simulink model "train_network"  (R2019a)
settings: Solver=VariableStepAuto  StartTime=0.0  StopTime=2400  RelTol=1e-3
values from neighbouring files (symbols this model uses):
  door_opening = [15 15 15 15 15 15 15]    [get_parameters.m]
  train_frequencies = struct    [get_parameters.m]
  travel_times = [ 0       60    0      0      0     0        0 ... (first row only)    [get_parameters.m]
undefined symbols (not defined in the file or in its folder): m, n
(part 1 of 2)
settings Model: SimulationMode=accelerator  OrderedModelArguments=off  Creator=Fredrik Rahm  LastModifiedBy=mawass

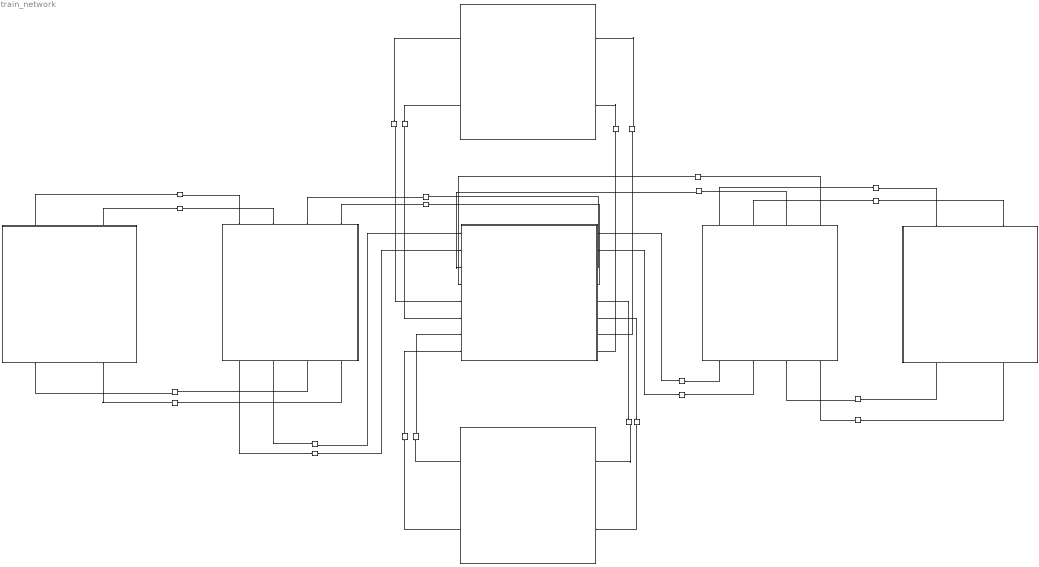
== system train_network ==
  Door signal delay1 : EntityServer  InputPortMessageModes=m  OutputPortMessageModes=m  Capacity=inf  ServiceTimeValue=travel_times(4,5)
  Signal delay10 : EntityServer  InputPortMessageModes=m  OutputPortMessageModes=m  Capacity=inf  ServiceTimeValue=travel_times(4,3)
  Signal delay11 : EntityServer  InputPortMessageModes=m  OutputPortMessageModes=m  Capacity=inf  ServiceTimeValue=travel_times(3,2)
  Signal delay12 : EntityServer  InputPortMessageModes=m  OutputPortMessageModes=m  Capacity=inf  ServiceTimeValue=travel_times(6,3)
  Signal delay14 : EntityServer  InputPortMessageModes=m  OutputPortMessageModes=m  Capacity=inf  ServiceTimeValue=travel_times(7,3)
  Signal delay2 : EntityServer  InputPortMessageModes=m  OutputPortMessageModes=m  Capacity=inf  ServiceTimeValue=travel_times(3,7)
  Signal delay3 : EntityServer  InputPortMessageModes=m  OutputPortMessageModes=m  Capacity=inf  ServiceTimeValue=travel_times(1,2)
  Signal delay4 : EntityServer  InputPortMessageModes=m  OutputPortMessageModes=m  Capacity=inf  ServiceTimeValue=travel_times(2,1)
  Signal delay5 : EntityServer  InputPortMessageModes=m  OutputPortMessageModes=m  Capacity=inf  ServiceTimeValue=travel_times(5,4)
  Signal delay6 : EntityServer  InputPortMessageModes=m  OutputPortMessageModes=m  Capacity=inf  ServiceTimeValue=travel_times(3,6)
  Signal delay8 : EntityServer  InputPortMessageModes=m  OutputPortMessageModes=m  Capacity=inf  ServiceTimeValue=travel_times(2,3)
  Signal delay9 : EntityServer  InputPortMessageModes=m  OutputPortMessageModes=m  Capacity=inf  ServiceTimeValue=travel_times(3,4)
  Station 1 : Subsystem
  Station 1. East. Travelling to Station 2. : EntityServer  InputPortMessageModes=m  OutputPortMessageModes=n,m  Capacity=train_cap  ServiceTimeValue=travel_times(1,2)  NumberEntitiesInBlock=on
      settings: OutputPortMap=o1,o9
  Station 2 : Subsystem
  Station 2. East. Travelling to Station 3. : EntityServer  InputPortMessageModes=m  OutputPortMessageModes=n,m  Capacity=train_cap  ServiceTimeValue=travel_times(2,3)  NumberEntitiesInBlock=on
      settings: OutputPortMap=o1,o9
  Station 2. West. Travelling to Station 1. : EntityServer  InputPortMessageModes=m  OutputPortMessageModes=n,m  Capacity=train_cap  ServiceTimeValue=travel_times(2,1)  NumberEntitiesInBlock=on
      settings: OutputPortMap=o1,o9
  Station 3 : Subsystem
  Station 3. East. Travelling to Station 4. : EntityServer  InputPortMessageModes=m  OutputPortMessageModes=n,m  Capacity=train_cap  ServiceTimeValue=travel_times(3,4)  NumberEntitiesInBlock=on
      settings: OutputPortMap=o1,o9
  Station 3. North. Travelling to Station 6. : EntityServer  InputPortMessageModes=m  OutputPortMessageModes=n,m  Capacity=train_cap  ServiceTimeValue=travel_times(3,6)  NumberEntitiesInBlock=on
      settings: OutputPortMap=o1,o9
  Station 3. West. Travelling to Station 2. : EntityServer  InputPortMessageModes=m  OutputPortMessageModes=n,m  Capacity=train_cap  ServiceTimeValue=travel_times(3,2)  NumberEntitiesInBlock=on
      settings: OutputPortMap=o1,o9
  Station 4 : Subsystem
  Station 4. East. Travelling to Station 5. : EntityServer  InputPortMessageModes=m  OutputPortMessageModes=n,m  Capacity=train_cap  ServiceTimeValue=travel_times(4,5)  NumberEntitiesInBlock=on
      settings: OutputPortMap=o1,o9
  Station 4. West. Travelling to Station 3. : EntityServer  InputPortMessageModes=m  OutputPortMessageModes=n,m  Capacity=train_cap  ServiceTimeValue=travel_times(4,3)  NumberEntitiesInBlock=on
      settings: OutputPortMap=o1,o9
  Station 5 : Subsystem
  Station 5. West. Travelling to Station 4. : EntityServer  InputPortMessageModes=m  OutputPortMessageModes=n,m  Capacity=train_cap  ServiceTimeValue=travel_times(5,4)  NumberEntitiesInBlock=on
      settings: OutputPortMap=o1,o9
  Station 6 : Subsystem
  Station 6. South. Travelling to Station 3. : EntityServer  InputPortMessageModes=m  OutputPortMessageModes=n,m  Capacity=1000  ServiceTimeValue=travel_times(6,3)  NumberEntitiesInBlock=on
      settings: OutputPortMap=o1,o9
  "Station 7 " : Subsystem
  Station 8. South. Travelling to Station 9. : EntityServer  InputPortMessageModes=m  OutputPortMessageModes=n,m  Capacity=train_cap  ServiceTimeValue=travel_times(3,7)  NumberEntitiesInBlock=on
      settings: OutputPortMap=o1,o9
  Station 9. North. Travelling to Station 8. : EntityServer  InputPortMessageModes=m  OutputPortMessageModes=n,m  Capacity=train_cap  ServiceTimeValue=travel_times(7,3)  NumberEntitiesInBlock=on
      settings: OutputPortMap=o1,o9
  wires:
  Station 4. East. Travelling to Station 5./2 -> Station 5/1(People in east)
  Door signal delay1/1 -> Station 5/2(Signal in east)
  Station 5/1(Train out west) -> Station 5. West. Travelling to Station 4./1
  Station 5/2(Signal out west) -> Signal delay5/1
  Station 3/2(Signal East out) -> Signal delay9/1
  Station 5. West. Travelling to Station 4./2 -> Station 4/3(Train in west)
  Signal delay5/1 -> Station 4/4(Signal in west)
  Station 4/1(People east) -> Station 4. East. Travelling to Station 5./1
  Station 4/2(Signal east) -> Door signal delay1/1
  Station 4/3(People west) -> Station 4. West. Travelling to Station 3./1
  Station 1. East. Travelling to Station 2./2 -> Station 2/1(People in east)
  Signal delay3/1 -> Station 2/2(Signal in east)
  Station 3/3(Train West out) -> Station 3. West. Travelling to Station 2./1
  Station 2/2(People out east) -> Station 2. East. Travelling to Station 3./1
  Station 2/3(People out west) -> Station 2. West. Travelling to Station 1./1
  Station 2/4(Signal out west) -> Signal delay4/1
  Station 2. West. Travelling to Station 1./2 -> Station 1/1(Train in west)
  Signal delay4/1 -> Station 1/2(Signal in west)
  Station 1/1(People east) -> Station 1. East. Travelling to Station 2./1
  Station 1/2(Signal East) -> Signal delay3/1
  Station 3/8(Signal North out) -> Signal delay6/1
  Station 8. South. Travelling to Station 9./2 -> "Station 7 "/1(People in south)
  Signal delay2/1 -> "Station 7 "/2(Signal in south)
  "Station 7 "/1(People out north) -> Station 9. North. Travelling to Station 8./1
  "Station 7 "/2(Signal out north) -> Signal delay14/1
  Station 3/7(Train North out) -> Station 3. North. Travelling to Station 6./1
  Station 2. East. Travelling to Station 3./2 -> Station 3/1(Train East in)
  Station 2/1(Signal out east) -> Signal delay8/1
  Signal delay8/1 -> Station 3/2(Signal East in)
  Signal delay9/1 -> Station 4/2(Signal in east)
  Station 3. East. Travelling to Station 4./2 -> Station 4/1(People in east)
  Station 3/1(Train East out) -> Station 3. East. Travelling to Station 4./1
  Station 4. West. Travelling to Station 3./2 -> Station 3/3(Train West in)
  Signal delay10/1 -> Station 3/4(Signal West in)
  Station 4/4(Signal west) -> Signal delay10/1
  Station 3. West. Travelling to Station 2./2 -> Station 2/3(People in west)
  Signal delay11/1 -> Station 2/4(Signal in west)
  Station 3/4(Signal West out) -> Signal delay11/1
  Signal delay12/1 -> Station 3/6(Signal South in)
  Station 6. South. Travelling to Station 3./2 -> Station 3/5(Train South in)
  Signal delay14/1 -> Station 3/8(Signal North in)
  Station 9. North. Travelling to Station 8./2 -> Station 3/7(Train North in)
  Station 3/5(Train South out) -> Station 8. South. Travelling to Station 9./1
  Station 3/6(Signal South out) -> Signal delay2/1
  Station 6/1(Train South) -> Station 6. South. Travelling to Station 3./1
  Station 6/2(Signal south) -> Signal delay12/1
  Signal delay6/1 -> Station 6/2(Signal north)
  Station 3. North. Travelling to Station 6./2 -> Station 6/1(Train north)

== system train_network/Station 1 ==
  Train in west : Inport
  Signal in west : Inport  Port=2
  Add : Sum
  Counting : EntityServer  InputPortMessageModes=m  OutputPortMessageModes=n,m  Capacity=inf  ServiceTimeSource=MATLAB action  ServiceTimeValue=1  ServiceTimeAction=|  NumberEntitiesInBlock=on
      | persistent rngInit;
      | if isempty(rngInit)
      |     seed = 12345;
      |     rng(seed);
      |     rngInit = true;
      | end
      | 
      | % Pattern: Gaussian (normal) distribution
      | % m: Mean, d: Standard deviation
      | m = 40; d = 8;
      | dt = m + d * randn;
      settings: OutputPortMap=o1,o9
  Entity Queue : EntityQueue  InputPortMessageModes=m  OutputPortMessageModes=m  Capacity=50  EntryAction=|
      | coder.extrinsic("get_param");
      | time = double(0);
      | time = get_param("train_network", "SimulationTime");
      | lifetime = time - entity.Timer;
      | 
      | coder.extrinsic("evalin");
      | evalin("base", sprintf("lifetimes_1(1,end+1) = %f; lifetimes_1(2,end) = %f;", lifetime, entity.StartStation));
      settings: OutputPortMap=o5
  Entity Terminator : EntityTerminator  InputPortMessageModes=m
  Station 1 - East : Subsystem
  Station 1 - West : Subsystem
  Station 1. People arriving. : EntityGenerator  OutputPortMessageModes=m  TimeSource=MATLAB action  IntergenerationTimeAction=|  GenerateAction=|  AttributeName=EndStation|Timer|StartStation  AttributeInitialValue=0|0|1  EntityType=Structured  EntityTypeName=Inbound
      | persistent rngInit;
      | if isempty(rngInit)
      |     seed = 173499;
      |     rng(seed);
      |     rngInit = true;
      | end
      | 
      | % Pattern: Exponential distribution
      | mu = lambda(1);
      | dt = -mu * log(1 - rand());
      | persistent rngInit;
      | if isempty(rngInit)
      |     seed = 12345;
      |     rng(seed);
      |     rngInit = true;
      | end
      | 
      | % Pattern: Arbitrary discrete distribution
      | % V: Value vector
      | % P: Probability vector
      | V = [1 2 3 4 5 6 7];
      | Ps = P(entity.StartStation,:);
      | entity.EndStation = randsample(V, 1, true, Ps);
      | 
      | coder.extrinsic("get_param");
      | entity.Timer = get_param("train_network", "SimulationTime");
  People east : Outport
  Signal East : Outport  Port=2
  wires:
  Train in west/1 -> Station 1 - West/1(Train in)
  Station 1 - East/2(Signal) -> Signal East/1
  Signal in west/1 -> Station 1 - West/2(Door control)
  Station 1. People arriving./1 -> Station 1 - East/1(Inport)
  Station 1 - East/1(Train) -> People east/1
  Counting/2 -> Entity Terminator/1
  Counting/1 -> Add/1
  Entity Queue/1 -> Counting/1
  Station 1 - West/1("Unboard ") -> Entity Queue/1
  Station 1 - East/3(Peopleplatform number) -> Add/2

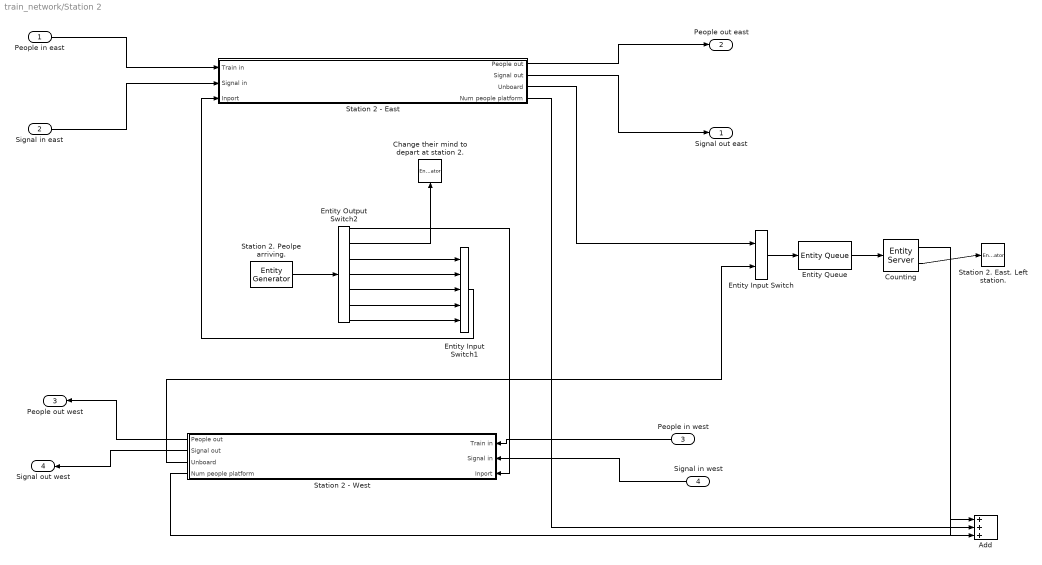
== system train_network/Station 2 ==
  People in east : Inport
  Signal in east : Inport  Port=2
  People in west : Inport  Port=3
  Signal in west : Inport  Port=4
  Add : Sum  Inputs=+++
  Change their mind to depart at station 2. : EntityTerminator  InputPortMessageModes=m
  Counting : EntityServer  InputPortMessageModes=m  OutputPortMessageModes=n,m  Capacity=inf  ServiceTimeSource=MATLAB action  ServiceTimeValue=1  ServiceTimeAction=|  NumberEntitiesInBlock=on
      | persistent rngInit;
      | if isempty(rngInit)
      |     seed = 12345;
      |     rng(seed);
      |     rngInit = true;
      | end
      | 
      | % Pattern: Gaussian (normal) distribution
      | % m: Mean, d: Standard deviation
      | m = 40; d = 8;
      | dt = m + d * randn;
      settings: OutputPortMap=o1,o9
  Entity Input Switch : EntityInputSwitch  InputPortMessageModes=m,m  OutputPortMessageModes=m
  Entity Input Switch1 : EntityInputSwitch  InputPortMessageModes=m,m,m,m,m  OutputPortMessageModes=m  NumberInputPorts=5
      settings: InputPortMap=u1,u2,u3,u4,u5
  Entity Output Switch2 : EntityOutputSwitch  InputPortMessageModes=m  OutputPortMessageModes=m,m,m,m,m,m,m  NumberOutputPorts=7  SwitchingCriterion=From attribute  SwitchAttributeName=EndStation
      settings: OutputPortMap=o0,o1,o2,o3,o4,o5,o6
  Entity Queue : EntityQueue  InputPortMessageModes=m  OutputPortMessageModes=m  Capacity=50  EntryAction=|
      | coder.extrinsic("get_param");
      | time = double(0);
      | time = get_param("train_network", "SimulationTime");
      | lifetime = time - entity.Timer;
      | 
      | coder.extrinsic("evalin");
      | evalin("base", sprintf("lifetimes_2(1,end+1) = %f; lifetimes_2(2,end) = %f;", lifetime, entity.StartStation));
      settings: OutputPortMap=o5
  Station 2 - East : Subsystem
  Station 2 - West : Subsystem
  Station 2. East. Left station. : EntityTerminator  InputPortMessageModes=m  NumberEntitiesArrived=on
      settings: OutputPortMap=o0
  Station 2. Peolpe arriving. : EntityGenerator  OutputPortMessageModes=m  TimeSource=MATLAB action  IntergenerationTimeAction=|  GenerateAction=|  AttributeName=EndStation|Timer|StartStation  AttributeInitialValue=0|0|2  EntityType=Structured  EntityTypeName=Inbound
      | persistent rngInit;
      | if isempty(rngInit)
      |     seed = 173499;
      |     rng(seed);
      |     rngInit = true;
      | end
      | 
      | % Pattern: Exponential distribution
      | mu = lambda(2);
      | dt = -mu * log(1 - rand());
      | persistent rngInit;
      | if isempty(rngInit)
      |     seed = 12345;
      |     rng(seed);
      |     rngInit = true;
      | end
      | 
      | % Pattern: Arbitrary discrete distribution
      | % V: Value vector
      | % P: Probability vector
      | V = [1 2 3 4 5 6 7];
      | Ps = P(entity.StartStation,:);
      | entity.EndStation = randsample(V, 1, true, Ps);
      | 
      | coder.extrinsic("get_param");
      | entity.Timer = get_param("train_network", "SimulationTime");
  Signal out east : Outport
  People out east : Outport  Port=2
  People out west : Outport  Port=3
  Signal out west : Outport  Port=4
  wires:
  Signal in west/1 -> Station 2 - West/2(Signal in)
  Entity Input Switch1/1 -> Station 2 - East/3(Inport)
  Entity Output Switch2/1 -> Station 2 - West/3(Inport)
  Station 2 - West/1(People out) -> People out west/1
  People in east/1 -> Station 2 - East/1(Train in)
  Station 2 - East/2(Signal out) -> Signal out east/1
  Station 2 - East/1(People out) -> People out east/1
  People in west/1 -> Station 2 - West/1(Train in)
  Station 2 - West/2(Signal out) -> Signal out west/1
  Signal in east/1 -> Station 2 - East/2(Signal in)
  Station 2. Peolpe arriving./1 -> Entity Output Switch2/1
  Entity Output Switch2/7 -> Entity Input Switch1/5
  Entity Output Switch2/6 -> Entity Input Switch1/4
  Entity Output Switch2/5 -> Entity Input Switch1/3
  Entity Output Switch2/4 -> Entity Input Switch1/2
  Entity Output Switch2/3 -> Entity Input Switch1/1
  Entity Output Switch2/2 -> Change their mind to depart at station 2./1
  Station 2 - East/3(Unboard) -> Entity Input Switch/1
  Station 2 - West/3(Unboard) -> Entity Input Switch/2
  Station 2 - West/4(Num people platform) -> Add/3
  Counting/2 -> Station 2. East. Left station./1
  Counting/1 -> Add/1
  Station 2 - East/4("Num people platform ") -> Add/2
  Entity Input Switch/1 -> Entity Queue/1
  Entity Queue/1 -> Counting/1

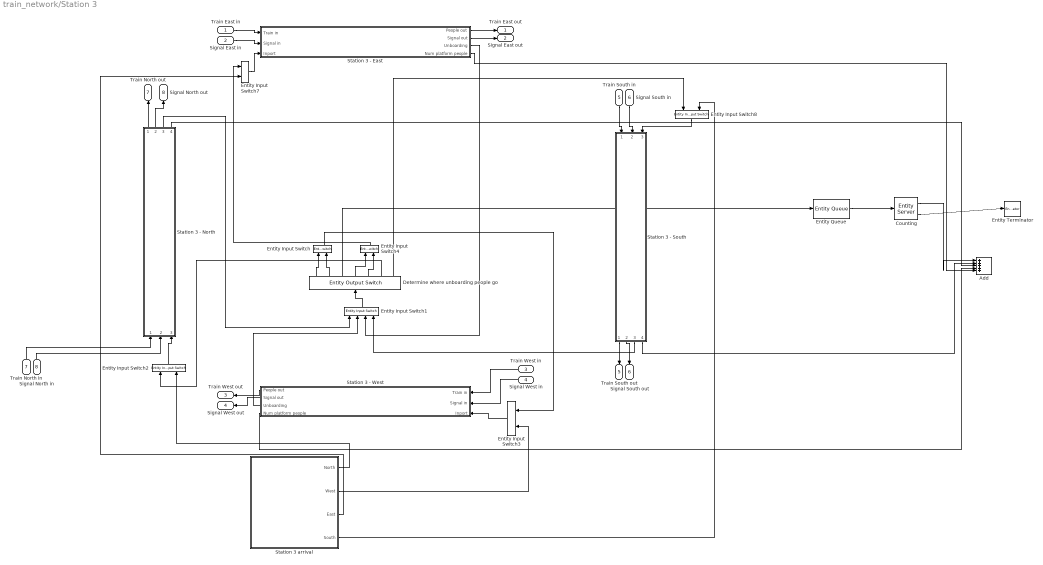
== system train_network/Station 3 ==
  Train East in : Inport
  Signal East in : Inport  Port=2
  Train West in : Inport  Port=3
  Signal West in : Inport  Port=4
  Train South in : Inport  Port=5
  Signal South in : Inport  Port=6
  Train North in : Inport  Port=7
  Signal North in : Inport  Port=8
  Add : Sum  Inputs=+++++
  Counting : EntityServer  InputPortMessageModes=m  OutputPortMessageModes=n,m  Capacity=inf  ServiceTimeSource=MATLAB action  ServiceTimeValue=1  ServiceTimeAction=|  NumberEntitiesInBlock=on
      | persistent rngInit;
      | if isempty(rngInit)
      |     seed = 12345;
      |     rng(seed);
      |     rngInit = true;
      | end
      | 
      | % Pattern: Gaussian (normal) distribution
      | % m: Mean, d: Standard deviation
      | m = 40; d = 8;
      | dt = m + d * randn;
      settings: OutputPortMap=o1,o9
  Determine where unboarding people go : EntityOutputSwitch  InputPortMessageModes=m  OutputPortMessageModes=m,m,m,m,m,m,m  NumberOutputPorts=7  SwitchingCriterion=From attribute  SwitchAttributeName=EndStation
      settings: OutputPortMap=o0,o1,o2,o3,o4,o5,o6
  Entity Input Switch{,2..4,7..8} (6 alike) : EntityInputSwitch  InputPortMessageModes=m,m  OutputPortMessageModes=m
  Entity Input Switch1 : EntityInputSwitch  InputPortMessageModes=m,m,m,m  OutputPortMessageModes=m  NumberInputPorts=4
      settings: InputPortMap=u1,u2,u3,u4
  Entity Queue : EntityQueue  InputPortMessageModes=m  OutputPortMessageModes=m  Capacity=50  EntryAction=|
      | coder.extrinsic("get_param");
      | time = double(0);
      | time = get_param("train_network", "SimulationTime");
      | lifetime = time - entity.Timer;
      | 
      | coder.extrinsic("evalin");
      | evalin("base", sprintf("lifetimes_3(1,end+1) = %f; lifetimes_3(2,end) = %f;", lifetime, entity.StartStation));
      settings: OutputPortMap=o5
  Entity Terminator : EntityTerminator  InputPortMessageModes=m
  Station 3 - East : Subsystem
  Station 3 - North : Subsystem
  Station 3 - South : Subsystem
  Station 3 - West : Subsystem
  Station 3 arrival : Subsystem
  Train East out : Outport
  Signal East out : Outport  Port=2
  Train West out : Outport  Port=3
  Signal West out : Outport  Port=4
  Train South out : Outport  Port=5
  Signal South out : Outport  Port=6
  Train North out : Outport  Port=7
  Signal North out : Outport  Port=8
  wires:
  Train East in/1 -> Station 3 - East/1(Train in)
  Station 3 - East/1(People out) -> Train East out/1
  Station 3 - East/2(Signal out) -> Signal East out/1
  Signal East in/1 -> Station 3 - East/2(Signal in)
  Station 3 - West/1(People out) -> Train West out/1
  Station 3 - West/2(Signal out) -> Signal West out/1
  Train West in/1 -> Station 3 - West/1(Train in)
  Signal West in/1 -> Station 3 - West/2(Signal in)
  Signal South in/1 -> Station 3 - South/2(Signal in)
  Train South in/1 -> Station 3 - South/1(Train in)
  Station 3 - South/2(Signal out) -> Signal South out/1
  Station 3 - South/1(People out) -> Train South out/1
  Signal North in/1 -> Station 3 - North/2(Signal in)
  Train North in/1 -> Station 3 - North/1(Train in)
  Station 3 - North/1(People out) -> Train North out/1
  Station 3 - North/2(Signal out) -> Signal North out/1
  Station 3 arrival/2(West) -> Entity Input Switch3/2
  Station 3 arrival/3(East) -> Entity Input Switch7/2
  Station 3 arrival/4(South) -> Entity Input Switch8/2
  Station 3 - North/3(Unboarding) -> Entity Input Switch1/1
  Station 3 - South/3(Unboarding) -> Entity Input Switch1/4
  Station 3 - West/3(Unboarding) -> Entity Input Switch1/2
  Station 3 - East/3(Unboarding) -> Entity Input Switch1/3
  Entity Input Switch2/1 -> Station 3 - North/3(Inport)
  Station 3 arrival/1(North) -> Entity Input Switch2/2
  Entity Input Switch1/1 -> Determine where unboarding people go/1
  Determine where unboarding people go/1 -> Entity Input Switch/1
  Determine where unboarding people go/2 -> Entity Input Switch/2
  Entity Input Switch3/1 -> Station 3 - West/3(Inport)
  Entity Input Switch/1 -> Entity Input Switch3/1
  Determine where unboarding people go/4 -> Entity Input Switch4/1
  Determine where unboarding people go/5 -> Entity Input Switch4/2
  Entity Input Switch7/1 -> Station 3 - East/3(Inport)
  Entity Input Switch4/1 -> Entity Input Switch7/1
  Entity Input Switch8/1 -> Station 3 - South/3(Inport)
  Determine where unboarding people go/6 -> Entity Input Switch2/1
  Determine where unboarding people go/7 -> Entity Input Switch8/1
  Counting/2 -> Entity Terminator/1
  Counting/1 -> Add/1
  Determine where unboarding people go/3 -> Entity Queue/1
  Entity Queue/1 -> Counting/1
  Station 3 - South/4(Num platform people) -> Add/2
  Station 3 - West/4(Num platform people) -> Add/4
  Station 3 - North/4(Num platform people) -> Add/3
  Station 3 - East/4(Num platform people) -> Add/5

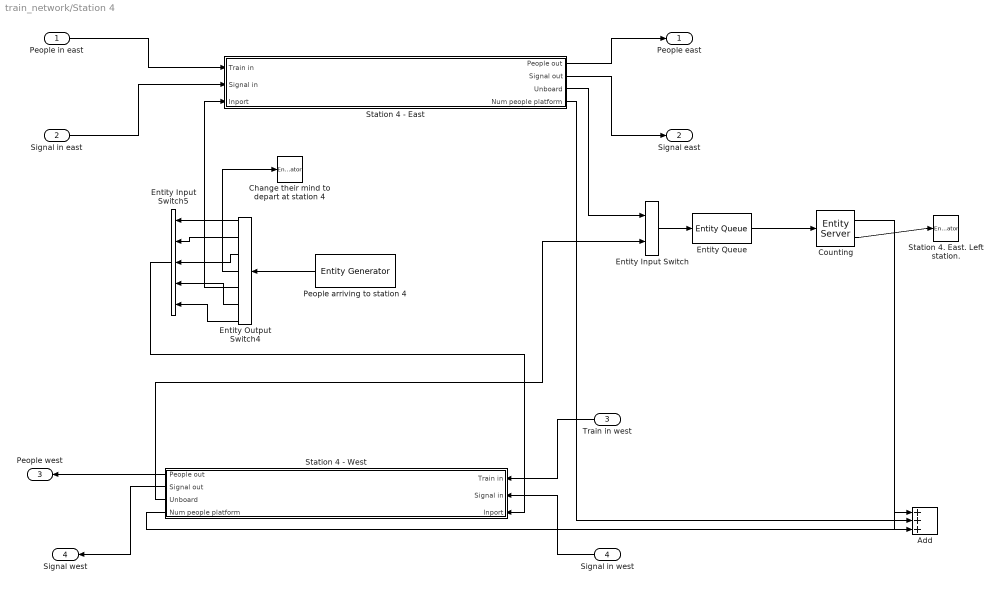
== system train_network/Station 4 ==
  People in east : Inport
  Signal in east : Inport  Port=2
  Train in west : Inport  Port=3
  Signal in west : Inport  Port=4
  Add : Sum  Inputs=+++
  Change their mind to depart at station 4 : EntityTerminator  InputPortMessageModes=m
  Counting : EntityServer  InputPortMessageModes=m  OutputPortMessageModes=n,m  Capacity=inf  ServiceTimeSource=MATLAB action  ServiceTimeValue=1  ServiceTimeAction=|  NumberEntitiesInBlock=on
      | persistent rngInit;
      | if isempty(rngInit)
      |     seed = 12345;
      |     rng(seed);
      |     rngInit = true;
      | end
      | 
      | % Pattern: Gaussian (normal) distribution
      | % m: Mean, d: Standard deviation
      | m = 40; d = 8;
      | dt = m + d * randn;
      settings: OutputPortMap=o1,o9
  Entity Input Switch : EntityInputSwitch  InputPortMessageModes=m,m  OutputPortMessageModes=m
  Entity Input Switch5 : EntityInputSwitch  InputPortMessageModes=m,m,m,m,m  OutputPortMessageModes=m  NumberInputPorts=5
      settings: InputPortMap=u1,u2,u3,u4,u5
  Entity Output Switch4 : EntityOutputSwitch  InputPortMessageModes=m  OutputPortMessageModes=m,m,m,m,m,m,m  NumberOutputPorts=7  SwitchingCriterion=From attribute  SwitchAttributeName=EndStation
      settings: OutputPortMap=o0,o1,o2,o3,o4,o5,o6
  Entity Queue : EntityQueue  InputPortMessageModes=m  OutputPortMessageModes=m  Capacity=50  EntryAction=|
      | coder.extrinsic("get_param");
      | time = double(0);
      | time = get_param("train_network", "SimulationTime");
      | lifetime = time - entity.Timer;
      | 
      | coder.extrinsic("evalin");
      | evalin("base", sprintf("lifetimes_4(1,end+1) = %f; lifetimes_4(2,end) = %f;", lifetime, entity.StartStation));
      settings: OutputPortMap=o5
  People arriving to station 4 : EntityGenerator  OutputPortMessageModes=m  TimeSource=MATLAB action  IntergenerationTimeAction=|  GenerateAction=|  AttributeName=EndStation|Timer|StartStation  AttributeInitialValue=0|1|4  EntityType=Structured  EntityTypeName=Inbound
      | persistent rngInit;
      | if isempty(rngInit)
      |     seed = 173499;
      |     rng(seed);
      |     rngInit = true;
      | end
      | 
      | % Pattern: Exponential distribution
      | mu = lambda(4);
      | dt = -mu * log(1 - rand());
      | persistent rngInit;
      | if isempty(rngInit)
      |     seed = 12345;
      |     rng(seed);
      |     rngInit = true;
      | end
      | 
      | % Pattern: Arbitrary discrete distribution
      | % V: Value vector
      | % P: Probability vector
      | V = [1 2 3 4 5 6 7];
      | Ps = P(entity.StartStation,:);
      | entity.EndStation = randsample(V, 1, true, Ps);
      | 
      | coder.extrinsic("get_param");
      | entity.Timer = get_param("train_network", "SimulationTime");
  Station 4 - East : Subsystem
  Station 4 - West : Subsystem
  Station 4. East. Left station. : EntityTerminator  InputPortMessageModes=m
  People east : Outport
  Signal east : Outport  Port=2
  People west : Outport  Port=3
  Signal west : Outport  Port=4
  wires:
  Entity Input Switch5/1 -> Station 4 - West/3(Inport)
  Signal in west/1 -> Station 4 - West/2(Signal in)
  Signal in east/1 -> Station 4 - East/2(Signal in)
  Entity Output Switch4/4 -> Change their mind to depart at station 4/1
  Station 4 - West/1(People out) -> People west/1
  Station 4 - West/2(Signal out) -> Signal west/1
  People in east/1 -> Station 4 - East/1(Train in)
  Entity Output Switch4/5 -> Station 4 - East/3(Inport)
  Station 4 - East/1(People out) -> People east/1
  Train in west/1 -> Station 4 - West/1(Train in)
  Station 4 - East/2(Signal out) -> Signal east/1
  People arriving to station 4/1 -> Entity Output Switch4/1
  Station 4 - East/3(Unboard) -> Entity Input Switch/1
  Station 4 - West/3(Unboard) -> Entity Input Switch/2
  Entity Output Switch4/1 -> Entity Input Switch5/1
  Entity Output Switch4/2 -> Entity Input Switch5/2
  Entity Output Switch4/3 -> Entity Input Switch5/3
  Entity Output Switch4/6 -> Entity Input Switch5/4
  Entity Output Switch4/7 -> Entity Input Switch5/5
  Entity Queue/1 -> Counting/1
  Counting/2 -> Station 4. East. Left station./1
  Counting/1 -> Add/1
  Entity Input Switch/1 -> Entity Queue/1
  Station 4 - West/4(Num people platform) -> Add/3
  Station 4 - East/4(Num people platform) -> Add/2

== system train_network/Station 5 ==
  People in east : Inport
  Signal in east : Inport  Port=2
  Add : Sum
  Counting : EntityServer  InputPortMessageModes=m  OutputPortMessageModes=n,m  Capacity=inf  ServiceTimeSource=MATLAB action  ServiceTimeValue=1  ServiceTimeAction=|  NumberEntitiesInBlock=on
      | persistent rngInit;
      | if isempty(rngInit)
      |     seed = 12345;
      |     rng(seed);
      |     rngInit = true;
      | end
      | 
      | % Pattern: Gaussian (normal) distribution
      | % m: Mean, d: Standard deviation
      | m = 40; d = 8;
      | dt = m + d * randn;
      settings: OutputPortMap=o1,o9
  Entity Queue : EntityQueue  InputPortMessageModes=m  OutputPortMessageModes=m  Capacity=50  EntryAction=|
      | coder.extrinsic("get_param");
      | time = double(0);
      | time = get_param("train_network", "SimulationTime");
      | lifetime = time - entity.Timer;
      | 
      | coder.extrinsic("evalin");
      | evalin("base", sprintf("lifetimes_5(1,end+1) = %f; lifetimes_5(2,end) = %f;", lifetime, entity.StartStation));
      settings: OutputPortMap=o5
  Entity Terminator : EntityTerminator  InputPortMessageModes=m
  People arriving to station 5. : EntityGenerator  OutputPortMessageModes=m  TimeSource=MATLAB action  IntergenerationTimeAction=|  GenerateAction=|  AttributeName=EndStation|Timer|StartStation  AttributeInitialValue=0|0|5  EntityType=Structured  EntityTypeName=Inbound
      | persistent rngInit;
      | if isempty(rngInit)
      |     seed = 173499;
      |     rng(seed);
      |     rngInit = true;
      | end
      | 
      | % Pattern: Exponential distribution
      | mu = lambda(5);
      | dt = -mu * log(1 - rand());
      | persistent rngInit;
      | if isempty(rngInit)
      |     seed = 12345;
      |     rng(seed);
      |     rngInit = true;
      | end
      | 
      | % Pattern: Arbitrary discrete distribution
      | % V: Value vector
      | % P: Probability vector
      | V = [1 2 3 4 5 6 7];
      | Ps = P(entity.StartStation,:);
      | entity.EndStation = randsample(V, 1, true, Ps);
      | 
      | coder.extrinsic("get_param");
      | entity.Timer = get_param("train_network", "SimulationTime");
  Station 5 - East : Subsystem
  Station 5 - West : Subsystem
  Train out west : Outport
  Signal out west : Outport  Port=2
  wires:
  Station 5 - West/2(Signal) -> Signal out west/1
  Station 5 - West/1(Train) -> Train out west/1
  Signal in east/1 -> Station 5 - East/2(Door control)
  People in east/1 -> Station 5 - East/1(Train in)
  Entity Queue/1 -> Counting/1
  Counting/2 -> Entity Terminator/1
  Counting/1 -> Add/1
  Station 5 - East/1("Unboard ") -> Entity Queue/1
  Station 5 - West/3(Platform number people) -> Add/2
  People arriving to station 5./1 -> Station 5 - West/1(Inport)

== system train_network/Station 6 ==
  Train north : Inport
  Signal north : Inport  Port=2
  Add : Sum
  Counting : EntityServer  InputPortMessageModes=m  OutputPortMessageModes=n,m  Capacity=inf  ServiceTimeSource=MATLAB action  ServiceTimeValue=1  ServiceTimeAction=|  NumberEntitiesInBlock=on
      | persistent rngInit;
      | if isempty(rngInit)
      |     seed = 12345;
      |     rng(seed);
      |     rngInit = true;
      | end
      | 
      | % Pattern: Gaussian (normal) distribution
      | % m: Mean, d: Standard deviation
      | m = 40; d = 8;
      | dt = m + d * randn;
      settings: OutputPortMap=o1,o9
  Entity Queue : EntityQueue  InputPortMessageModes=m  OutputPortMessageModes=m  Capacity=50  EntryAction=|
      | coder.extrinsic("get_param");
      | time = double(0);
      | time = get_param("train_network", "SimulationTime");
      | lifetime = time - entity.Timer;
      | 
      | coder.extrinsic("evalin");
      | evalin("base", sprintf("lifetimes_6(1,end+1) = %f; lifetimes_6(2,end) = %f;", lifetime, entity.StartStation));
      settings: OutputPortMap=o5
  Entity Terminator : EntityTerminator  InputPortMessageModes=m
  People arriving to station 6. : EntityGenerator  OutputPortMessageModes=m  TimeSource=MATLAB action  IntergenerationTimeAction=|  GenerateAction=|  AttributeName=EndStation|Timer|StartStation  AttributeInitialValue=0|0|6  EntityType=Structured  EntityTypeName=Inbound
      | persistent rngInit;
      | if isempty(rngInit)
      |     seed = 173499;
      |     rng(seed);
      |     rngInit = true;
      | end
      | 
      | % Pattern: Exponential distribution
      | mu = lambda(6);
      | dt = -mu * log(1 - rand());
      | persistent rngInit;
      | if isempty(rngInit)
      |     seed = 12345;
      |     rng(seed);
      |     rngInit = true;
      | end
      | 
      | % Pattern: Arbitrary discrete distribution
      | % V: Value vector
      | % P: Probability vector
      | V = [1 2 3 4 5 6 7];
      | Ps = P(entity.StartStation,:);
      | entity.EndStation = randsample(V, 1, true, Ps);
      | 
      | coder.extrinsic("get_param");
      | entity.Timer = get_param("train_network", "SimulationTime");
  Station 6 - North : Subsystem
  Station 6 - South : Subsystem
  Train South : Outport
  Signal south : Outport  Port=2
  wires:
  People arriving to station 6./1 -> Station 6 - South/1(Inport)
  Station 6 - South/2(Signal) -> Signal south/1
  Station 6 - South/1(Train) -> Train South/1
  Signal north/1 -> Station 6 - North/2(Door control)
  Train north/1 -> Station 6 - North/1(Train in)
  Counting/2 -> Entity Terminator/1
  Counting/1 -> Add/1
  Station 6 - North/1(Unboard) -> Entity Queue/1
  Entity Queue/1 -> Counting/1
  Station 6 - South/3("People on platform ") -> Add/2

== system train_network/Station 7  ==
  People in south : Inport
  Signal in south : Inport  Port=2
  Add : Sum
  Counting : EntityServer  InputPortMessageModes=m  OutputPortMessageModes=n,m  Capacity=inf  ServiceTimeSource=MATLAB action  ServiceTimeValue=1  ServiceTimeAction=|  NumberEntitiesInBlock=on
      | persistent rngInit;
      | if isempty(rngInit)
      |     seed = 12345;
      |     rng(seed);
      |     rngInit = true;
      | end
      | 
      | % Pattern: Gaussian (normal) distribution
      | % m: Mean, d: Standard deviation
      | m = 40; d = 8;
      | dt = m + d * randn;
      settings: OutputPortMap=o1,o9
  Entity Queue : EntityQueue  InputPortMessageModes=m  OutputPortMessageModes=m  Capacity=50  EntryAction=|
      | coder.extrinsic("get_param");
      | time = double(0);
      | time = get_param("train_network", "SimulationTime");
      | lifetime = time - entity.Timer;
      | 
      | coder.extrinsic("evalin");
      | evalin("base", sprintf("lifetimes_7(1,end+1) = %f; lifetimes_7(2,end) = %f;", lifetime, entity.StartStation));
      settings: OutputPortMap=o5
  Entity Terminator : EntityTerminator  InputPortMessageModes=m
  People arriving to station 7 : EntityGenerator  OutputPortMessageModes=m  TimeSource=MATLAB action  IntergenerationTimeAction=|  GenerateAction=|  AttributeName=EndStation|Timer|StartStation  AttributeInitialValue=0|0|7  EntityType=Structured  EntityTypeName=Inbound
      | persistent rngInit;
      | if isempty(rngInit)
      |     seed = 173499;
      |     rng(seed);
      |     rngInit = true;
      | end
      | 
      | % Pattern: Exponential distribution
      | mu = lambda(7);
      | dt = -mu * log(1 - rand());
      | persistent rngInit;
      | if isempty(rngInit)
      |     seed = 12345;
      |     rng(seed);
      |     rngInit = true;
      | end
      | 
      | % Pattern: Arbitrary discrete distribution
      | % V: Value vector
      | % P: Probability vector
      | V = [1 2 3 4 5 6 7];
      | Ps = P(entity.StartStation,:);
      | entity.EndStation = randsample(V, 1, true, Ps);
      | 
      | coder.extrinsic("get_param");
      | entity.Timer = get_param("train_network", "SimulationTime");
  Station 7 - North : Subsystem
  Station 7 - South : Subsystem
  People out north : Outport
  Signal out north : Outport  Port=2
  wires:
  Signal in south/1 -> Station 7 - South/2(Door control)
  Station 7 - North/2(Signal) -> Signal out north/1
  Station 7 - North/1(Train) -> People out north/1
  People arriving to station 7/1 -> Station 7 - North/1(Inport)
  People in south/1 -> Station 7 - South/1(Train in)
  Counting/2 -> Entity Terminator/1
  Station 7 - South/1(Out1) -> Entity Queue/1
  Entity Queue/1 -> Counting/1
  Counting/1 -> Add/2
  Station 7 - North/3("Num people platform ") -> Add/1

== system train_network/Station 1/Station 1 - East ==
  Inport : Inport
  Departure blocking : EntityGate  InputPortMessageModes=m,m  OutputPortMessageModes=m
  Door controller : Subsystem
  "Station 1, East Train arrives1" : EntityGate  InputPortMessageModes=m,m  OutputPortMessageModes=m
  Station 1. East. People in train while boarding. : EntityServer  InputPortMessageModes=m  OutputPortMessageModes=m  Capacity=train_cap  ServiceTimeValue=0
  Station 1. East. Platform. : EntityQueue  InputPortMessageModes=m  OutputPortMessageModes=n,m  Capacity=inf  NumberEntitiesInBlock=on
      settings: OutputPortMap=o1,o5
  Train : Outport
  Signal : Outport  Port=2
  Peopleplatform number : Outport  Port=3
  wires:
  Station 1. East. Platform./2 -> "Station 1, East Train arrives1"/2
  "Station 1, East Train arrives1"/1 -> Station 1. East. People in train while boarding./1
  Station 1. East. People in train while boarding./1 -> Departure blocking/2
  Departure blocking/1 -> Train/1
  Door controller/1(Next station) -> Signal/1
  Door controller/2(Departure) -> Departure blocking/1
  Door controller/3(Train door) -> "Station 1, East Train arrives1"/1
  Inport/1 -> Station 1. East. Platform./1
  Station 1. East. Platform./1 -> Peopleplatform number/1

== system train_network/Station 1/Station 1 - West ==
  Train in : Inport
  Door control : Inport  Port=2
  " " : EntityGate  InputPortMessageModes=m,m  OutputPortMessageModes=m
  "Unboard " : Outport
  wires:
  Door control/1 -> " "/1
  Train in/1 -> " "/2
  " "/1 -> "Unboard "/1

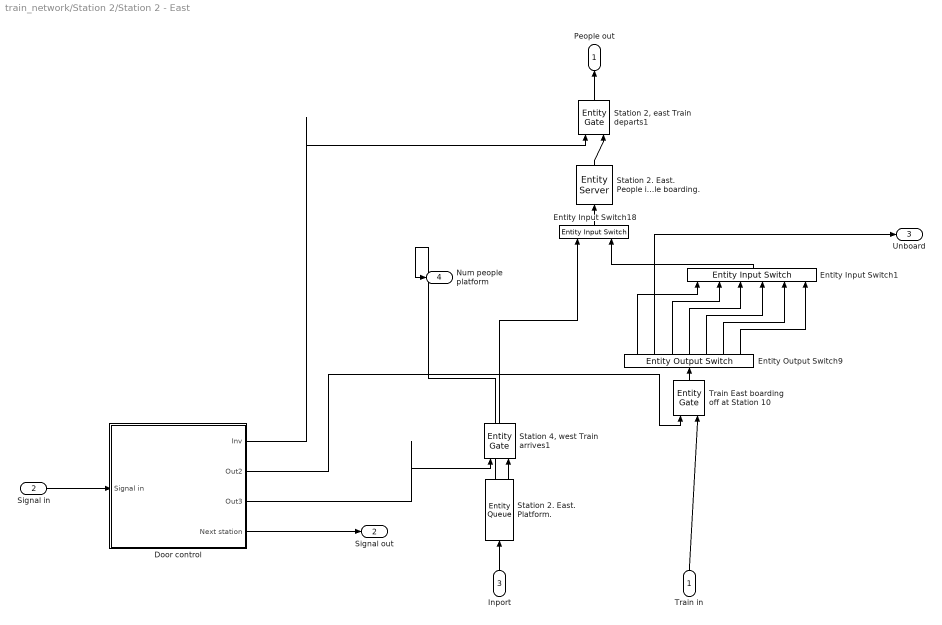
== system train_network/Station 2/Station 2 - East ==
  Train in : Inport
  Signal in : Inport  Port=2
  Inport : Inport  Port=3
  Door control : Subsystem
  Entity Input Switch1 : EntityInputSwitch  InputPortMessageModes=m,m,m,m,m,m  OutputPortMessageModes=m  NumberInputPorts=6
      settings: InputPortMap=u1,u2,u3,u4,u5,u6
  Entity Input Switch18 : EntityInputSwitch  InputPortMessageModes=m,m  OutputPortMessageModes=m
  Entity Output Switch9 : EntityOutputSwitch  InputPortMessageModes=m  OutputPortMessageModes=m,m,m,m,m,m,m  NumberOutputPorts=7  SwitchingCriterion=From attribute  SwitchAttributeName=EndStation
      settings: OutputPortMap=o0,o1,o2,o3,o4,o5,o6
  "Station 2, east Train departs1" : EntityGate  InputPortMessageModes=m,m  OutputPortMessageModes=m
  Station 2. East. People in train while boarding. : EntityServer  InputPortMessageModes=m  OutputPortMessageModes=m  Capacity=train_cap  ServiceTimeValue=0
  "Station 2. East. Platform. " : EntityQueue  InputPortMessageModes=m  OutputPortMessageModes=n,m  Capacity=inf  NumberEntitiesInBlock=on
      settings: OutputPortMap=o1,o5
  "Station 4, west Train arrives1" : EntityGate  InputPortMessageModes=m,m  OutputPortMessageModes=m
  Train East boarding off at Station 10 : EntityGate  InputPortMessageModes=m,m  OutputPortMessageModes=m
  People out : Outport
  Signal out : Outport  Port=2
  Unboard : Outport  Port=3
  "Num people platform " : Outport  Port=4
  wires:
  Train East boarding off at Station 10/1 -> Entity Output Switch9/1
  Inport/1 -> "Station 2. East. Platform. "/1
  Entity Input Switch18/1 -> Station 2. East. People in train while boarding./1
  Station 2. East. People in train while boarding./1 -> "Station 2, east Train departs1"/2
  Train in/1 -> Train East boarding off at Station 10/2
  "Station 2, east Train departs1"/1 -> People out/1
  "Station 2. East. Platform. "/2 -> "Station 4, west Train arrives1"/2
  Entity Output Switch9/1 -> Entity Input Switch1/1
  Entity Output Switch9/2 -> Unboard/1
  "Station 4, west Train arrives1"/1 -> Entity Input Switch18/1
  Door control/1(Inv) -> "Station 2, east Train departs1"/1
  Signal in/1 -> Door control/1(Signal in)
  Door control/4(Next station) -> Signal out/1
  Door control/2(Out2) -> Train East boarding off at Station 10/1
  Door control/3(Out3) -> "Station 4, west Train arrives1"/1
  Entity Output Switch9/3 -> Entity Input Switch1/2
  Entity Output Switch9/4 -> Entity Input Switch1/3
  Entity Output Switch9/5 -> Entity Input Switch1/4
  Entity Output Switch9/6 -> Entity Input Switch1/5
  Entity Output Switch9/7 -> Entity Input Switch1/6
  Entity Input Switch1/1 -> Entity Input Switch18/2
  "Station 2. East. Platform. "/1 -> "Num people platform "/1

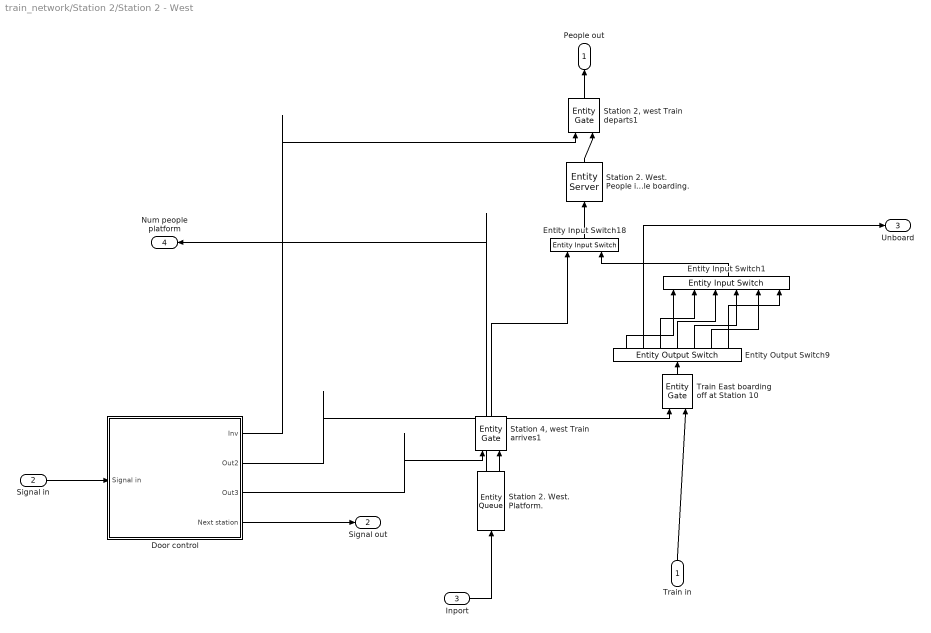
== system train_network/Station 2/Station 2 - West ==
  Train in : Inport
  Signal in : Inport  Port=2
  Inport : Inport  Port=3
  Door control : Subsystem
  Entity Input Switch1 : EntityInputSwitch  InputPortMessageModes=m,m,m,m,m,m  OutputPortMessageModes=m  NumberInputPorts=6
      settings: InputPortMap=u1,u2,u3,u4,u5,u6
  Entity Input Switch18 : EntityInputSwitch  InputPortMessageModes=m,m  OutputPortMessageModes=m
  Entity Output Switch9 : EntityOutputSwitch  InputPortMessageModes=m  OutputPortMessageModes=m,m,m,m,m,m,m  NumberOutputPorts=7  SwitchingCriterion=From attribute  SwitchAttributeName=EndStation
      settings: OutputPortMap=o0,o1,o2,o3,o4,o5,o6
  "Station 2, west Train departs1" : EntityGate  InputPortMessageModes=m,m  OutputPortMessageModes=m
  Station 2. West. People in train while boarding. : EntityServer  InputPortMessageModes=m  OutputPortMessageModes=m  Capacity=train_cap  ServiceTimeValue=0
  Station 2. West. Platform. : EntityQueue  InputPortMessageModes=m  OutputPortMessageModes=n,m  Capacity=inf  NumberEntitiesInBlock=on
      settings: OutputPortMap=o1,o5
  "Station 4, west Train arrives1" : EntityGate  InputPortMessageModes=m,m  OutputPortMessageModes=m
  Train East boarding off at Station 10 : EntityGate  InputPortMessageModes=m,m  OutputPortMessageModes=m
  People out : Outport
  Signal out : Outport  Port=2
  Unboard : Outport  Port=3
  Num people platform : Outport  Port=4
  wires:
  Inport/1 -> Station 2. West. Platform./1
  Entity Input Switch18/1 -> Station 2. West. People in train while boarding./1
  Station 2. West. People in train while boarding./1 -> "Station 2, west Train departs1"/2
  Train in/1 -> Train East boarding off at Station 10/2
  "Station 2, west Train departs1"/1 -> People out/1
  Station 2. West. Platform./2 -> "Station 4, west Train arrives1"/2
  "Station 4, west Train arrives1"/1 -> Entity Input Switch18/1
  Door control/1(Inv) -> "Station 2, west Train departs1"/1
  Signal in/1 -> Door control/1(Signal in)
  Door control/4(Next station) -> Signal out/1
  Door control/2(Out2) -> Train East boarding off at Station 10/1
  Door control/3(Out3) -> "Station 4, west Train arrives1"/1
  Entity Output Switch9/6 -> Entity Input Switch1/5
  Entity Output Switch9/1 -> Entity Input Switch1/1
  Entity Output Switch9/4 -> Entity Input Switch1/3
  Entity Input Switch1/1 -> Entity Input Switch18/2
  Entity Output Switch9/5 -> Entity Input Switch1/4
  Entity Output Switch9/3 -> Entity Input Switch1/2
  Entity Output Switch9/7 -> Entity Input Switch1/6
  Train East boarding off at Station 10/1 -> Entity Output Switch9/1
  Entity Output Switch9/2 -> Unboard/1
  Station 2. West. Platform./1 -> Num people platform/1

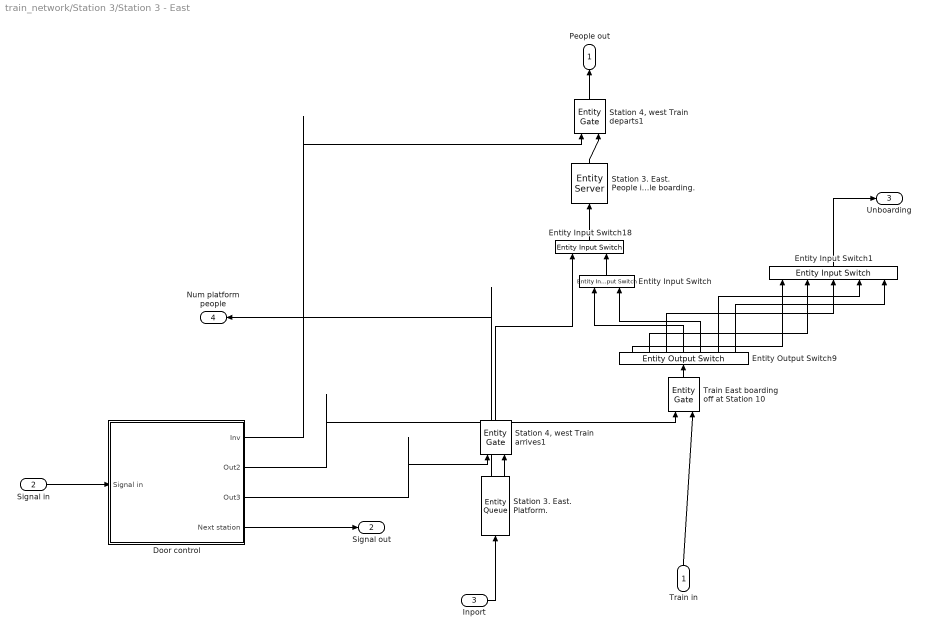
== system train_network/Station 3/Station 3 - East ==
  Train in : Inport
  Signal in : Inport  Port=2
  Inport : Inport  Port=3
  Door control : Subsystem
  Entity Input Switch : EntityInputSwitch  InputPortMessageModes=m,m  OutputPortMessageModes=m
  Entity Input Switch1 : EntityInputSwitch  InputPortMessageModes=m,m,m,m,m  OutputPortMessageModes=m  NumberInputPorts=5
      settings: InputPortMap=u1,u2,u3,u4,u5
  Entity Input Switch18 : EntityInputSwitch  InputPortMessageModes=m,m  OutputPortMessageModes=m
  Entity Output Switch9 : EntityOutputSwitch  InputPortMessageModes=m  OutputPortMessageModes=m,m,m,m,m,m,m  NumberOutputPorts=7  SwitchingCriterion=From attribute  SwitchAttributeName=EndStation
      settings: OutputPortMap=o0,o1,o2,o3,o4,o5,o6
  Station 3. East. People in train while boarding. : EntityServer  InputPortMessageModes=m  OutputPortMessageModes=m  Capacity=train_cap  ServiceTimeValue=0
  Station 3. East. Platform. : EntityQueue  InputPortMessageModes=m  OutputPortMessageModes=n,m  Capacity=inf  NumberEntitiesInBlock=on
      settings: OutputPortMap=o1,o5
  "Station 4, west Train departs1" : EntityGate  InputPortMessageModes=m,m  OutputPortMessageModes=m
  "Station 4, west Train arrives1" : EntityGate  InputPortMessageModes=m,m  OutputPortMessageModes=m
  Train East boarding off at Station 10 : EntityGate  InputPortMessageModes=m,m  OutputPortMessageModes=m
  People out : Outport
  Signal out : Outport  Port=2
  Unboarding : Outport  Port=3
  Num platform people : Outport  Port=4
  wires:
  Inport/1 -> Station 3. East. Platform./1
  Entity Input Switch18/1 -> Station 3. East. People in train while boarding./1
  Station 3. East. People in train while boarding./1 -> "Station 4, west Train departs1"/2
  Train in/1 -> Train East boarding off at Station 10/2
  "Station 4, west Train departs1"/1 -> People out/1
  Station 3. East. Platform./2 -> "Station 4, west Train arrives1"/2
  "Station 4, west Train arrives1"/1 -> Entity Input Switch18/1
  Door control/1(Inv) -> "Station 4, west Train departs1"/1
  Signal in/1 -> Door control/1(Signal in)
  Door control/4(Next station) -> Signal out/1
  Door control/2(Out2) -> Train East boarding off at Station 10/1
  Door control/3(Out3) -> "Station 4, west Train arrives1"/1
  Train East boarding off at Station 10/1 -> Entity Output Switch9/1
  Entity Input Switch/1 -> Entity Input Switch18/2
  Entity Output Switch9/4 -> Entity Input Switch/1
  Entity Output Switch9/5 -> Entity Input Switch/2
  Entity Output Switch9/1 -> Entity Input Switch1/1
  Entity Output Switch9/2 -> Entity Input Switch1/2
  Entity Output Switch9/3 -> Entity Input Switch1/3
  Entity Output Switch9/6 -> Entity Input Switch1/4
  Entity Output Switch9/7 -> Entity Input Switch1/5
  Entity Input Switch1/1 -> Unboarding/1
  Station 3. East. Platform./1 -> Num platform people/1

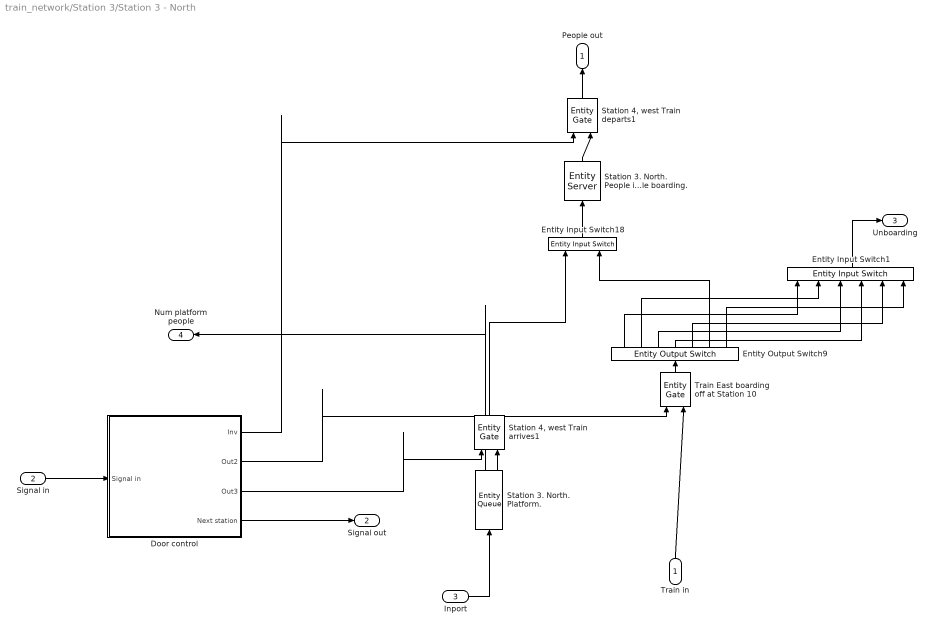
== system train_network/Station 3/Station 3 - North ==
  Train in : Inport
  Signal in : Inport  Port=2
  Inport : Inport  Port=3
  Door control : Subsystem
  Entity Input Switch1 : EntityInputSwitch  InputPortMessageModes=m,m,m,m,m,m  OutputPortMessageModes=m  NumberInputPorts=6
      settings: InputPortMap=u1,u2,u3,u4,u5,u6
  Entity Input Switch18 : EntityInputSwitch  InputPortMessageModes=m,m  OutputPortMessageModes=m
  Entity Output Switch9 : EntityOutputSwitch  InputPortMessageModes=m  OutputPortMessageModes=m,m,m,m,m,m,m  NumberOutputPorts=7  SwitchingCriterion=From attribute  SwitchAttributeName=EndStation
      settings: OutputPortMap=o0,o1,o2,o3,o4,o5,o6
  Station 3. North. People in train while boarding. : EntityServer  InputPortMessageModes=m  OutputPortMessageModes=m  Capacity=train_cap  ServiceTimeValue=0
  Station 3. North. Platform. : EntityQueue  InputPortMessageModes=m  OutputPortMessageModes=n,m  Capacity=inf  NumberEntitiesInBlock=on
      settings: OutputPortMap=o1,o5
  "Station 4, west Train departs1" : EntityGate  InputPortMessageModes=m,m  OutputPortMessageModes=m
  "Station 4, west Train arrives1" : EntityGate  InputPortMessageModes=m,m  OutputPortMessageModes=m
  Train East boarding off at Station 10 : EntityGate  InputPortMessageModes=m,m  OutputPortMessageModes=m
  People out : Outport
  Signal out : Outport  Port=2
  Unboarding : Outport  Port=3
  Num platform people : Outport  Port=4
  wires:
  Inport/1 -> Station 3. North. Platform./1
  Entity Input Switch18/1 -> Station 3. North. People in train while boarding./1
  Station 3. North. People in train while boarding./1 -> "Station 4, west Train departs1"/2
  Train in/1 -> Train East boarding off at Station 10/2
  "Station 4, west Train departs1"/1 -> People out/1
  Station 3. North. Platform./2 -> "Station 4, west Train arrives1"/2
  "Station 4, west Train arrives1"/1 -> Entity Input Switch18/1
  Door control/1(Inv) -> "Station 4, west Train departs1"/1
  Signal in/1 -> Door control/1(Signal in)
  Door control/4(Next station) -> Signal out/1
  Door control/2(Out2) -> Train East boarding off at Station 10/1
  Door control/3(Out3) -> "Station 4, west Train arrives1"/1
  Train East boarding off at Station 10/1 -> Entity Output Switch9/1
  Entity Output Switch9/6 -> Entity Input Switch18/2
  Entity Input Switch1/1 -> Unboarding/1
  Entity Output Switch9/1 -> Entity Input Switch1/1
  Entity Output Switch9/2 -> Entity Input Switch1/2
  Entity Output Switch9/3 -> Entity Input Switch1/3
  Entity Output Switch9/4 -> Entity Input Switch1/4
  Entity Output Switch9/5 -> Entity Input Switch1/5
  Entity Output Switch9/7 -> Entity Input Switch1/6
  Station 3. North. Platform./1 -> Num platform people/1

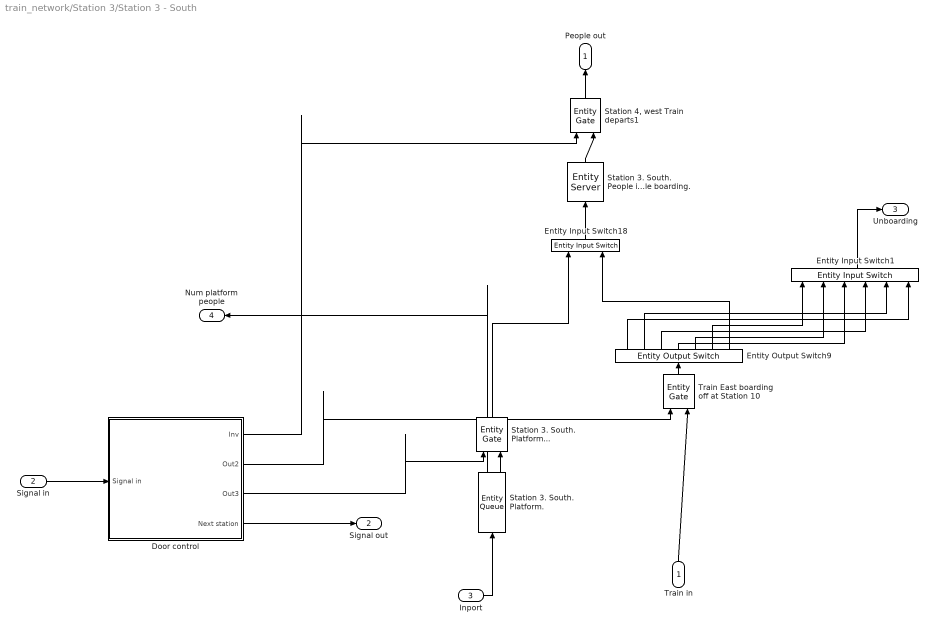
== system train_network/Station 3/Station 3 - South ==
  Train in : Inport
  Signal in : Inport  Port=2
  Inport : Inport  Port=3
  Door control : Subsystem
  Entity Input Switch1 : EntityInputSwitch  InputPortMessageModes=m,m,m,m,m,m  OutputPortMessageModes=m  NumberInputPorts=6
      settings: InputPortMap=u1,u2,u3,u4,u5,u6
  Entity Input Switch18 : EntityInputSwitch  InputPortMessageModes=m,m  OutputPortMessageModes=m
  Entity Output Switch9 : EntityOutputSwitch  InputPortMessageModes=m  OutputPortMessageModes=m,m,m,m,m,m,m  NumberOutputPorts=7  SwitchingCriterion=From attribute  SwitchAttributeName=EndStation
      settings: OutputPortMap=o0,o1,o2,o3,o4,o5,o6
  Station 3. South. People in train while boarding. : EntityServer  InputPortMessageModes=m  OutputPortMessageModes=m  Capacity=train_cap  ServiceTimeValue=0
  Station 3. South. Platform. : EntityQueue  InputPortMessageModes=m  OutputPortMessageModes=n,m  Capacity=inf  NumberEntitiesInBlock=on
      settings: OutputPortMap=o1,o5
  Station 3. South. Platform... : EntityGate  InputPortMessageModes=m,m  OutputPortMessageModes=m
  "Station 4, west Train departs1" : EntityGate  InputPortMessageModes=m,m  OutputPortMessageModes=m
  Train East boarding off at Station 10 : EntityGate  InputPortMessageModes=m,m  OutputPortMessageModes=m
  People out : Outport
  Signal out : Outport  Port=2
  Unboarding : Outport  Port=3
  Num platform people : Outport  Port=4
  wires:
  Inport/1 -> Station 3. South. Platform./1
  Entity Input Switch18/1 -> Station 3. South. People in train while boarding./1
  Station 3. South. People in train while boarding./1 -> "Station 4, west Train departs1"/2
  Train in/1 -> Train East boarding off at Station 10/2
  "Station 4, west Train departs1"/1 -> People out/1
  Station 3. South. Platform./2 -> Station 3. South. Platform.../2
  Station 3. South. Platform.../1 -> Entity Input Switch18/1
  Door control/1(Inv) -> "Station 4, west Train departs1"/1
  Signal in/1 -> Door control/1(Signal in)
  Door control/4(Next station) -> Signal out/1
  Door control/2(Out2) -> Train East boarding off at Station 10/1
  Door control/3(Out3) -> Station 3. South. Platform.../1
  Train East boarding off at Station 10/1 -> Entity Output Switch9/1
  Entity Output Switch9/7 -> Entity Input Switch18/2
  Entity Input Switch1/1 -> Unboarding/1
  Entity Output Switch9/6 -> Entity Input Switch1/1
  Entity Output Switch9/5 -> Entity Input Switch1/2
  Entity Output Switch9/4 -> Entity Input Switch1/3
  Entity Output Switch9/3 -> Entity Input Switch1/4
  Entity Output Switch9/2 -> Entity Input Switch1/5
  Entity Output Switch9/1 -> Entity Input Switch1/6
  Station 3. South. Platform./1 -> Num platform people/1
